simulink model "test1"  (R2014a)
settings: Solver=FixedStepDiscrete  StartTime=0.0  StopTime=10  RelTol=1e-3
InitFcn:
  | clear;
  | Pulse.clearPulses();
  | initPulse  = Pulse([]);
  | initPulseID = initPulse.ID;
  | inputsignal = zeros(10,1);
  | inputsignal(1) = initPulseID;
libraries: BlockLib x2, dspsrcs4 x1
settings Model: Creator=kunalmenda  LastModifiedBy=kunalmenda

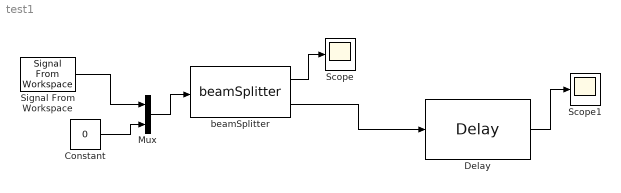
== system test1 ==
  Constant : Constant  Value=0
  Delay : BlockLib/Delay
  Mux : Mux  Inputs=2
  Scope : Scope
  Scope1 : Scope
  Signal From Workspace : dspsrcs4/Signal From Workspace  X=inputsignal  Ts=1  nsamps=1  OutputAfterFinalValue=Setting to zero  ignoreOrWarnInputAndFrameLengths=off
  "beamSplitter " : BlockLib/beamSplitter 
  wires:
  "beamSplitter "/1 -> Scope/1
  Signal From Workspace/1 -> Mux/1
  Mux/1 -> "beamSplitter "/1
  Constant/1 -> Mux/2
  "beamSplitter "/2 -> Delay/1
  Delay/1 -> Scope1/1
